simulink library "mat_3x3"  (R2020b)
settings: Solver=VariableStepAuto  StartTime=0.0  StopTime=10.0  RelTol=1e-3
settings Model: Creator=whitehole  LastModifiedBy=whitehole

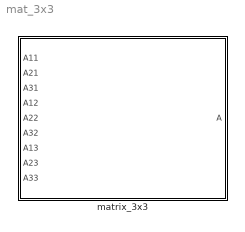
== system mat_3x3 ==
  matrix_3x3 : Subsystem

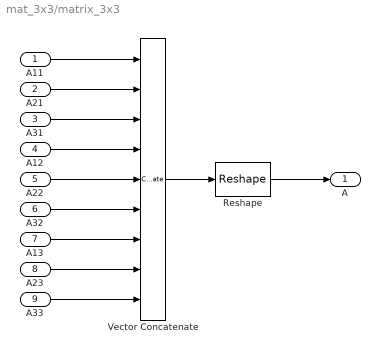
== system mat_3x3/matrix_3x3 ==
  A11 : Inport
  A21 : Inport  Port=2
  A31 : Inport  Port=3
  A12 : Inport  Port=4
  A22 : Inport  Port=5
  A32 : Inport  Port=6
  A13 : Inport  Port=7
  A23 : Inport  Port=8
  A33 : Inport  Port=9
  Reshape : Reshape  OutputDimensionality=Customize  OutputDimensions=[3,3]
  Vector Concatenate : Concatenate  NumInputs=9
  A : Outport
  wires:
  A23/1 -> Vector Concatenate/8
  A33/1 -> Vector Concatenate/9
  A22/1 -> Vector Concatenate/5
  Reshape/1 -> A/1
  A12/1 -> Vector Concatenate/4
  Vector Concatenate/1 -> Reshape/1
  A13/1 -> Vector Concatenate/7
  A11/1 -> Vector Concatenate/1
  A32/1 -> Vector Concatenate/6
  A31/1 -> Vector Concatenate/3
  A21/1 -> Vector Concatenate/2
